simulink model "IonSatSimulationF_UKF"  (R2020b)
settings: Solver=ode3  StartTime=0.0  StopTime=t_sim  FixedStep=TimeStep  MaxStep=30  MinStep=.1  RelTol=1e-3
model workspace (MAT data in the model file):
  repartition_matrix : Simulink.Parameter (value not decoded)
  wheel_number : Simulink.Parameter (value not decoded)
values from neighbouring files (symbols this model uses):
  controller = 1    [Scenario1_Monte_Carlo.m]    (also in main_ADCS_v2.m)
  K = [0.00053417  0  0  0.0070506  0  0 ... (first row only)    [Full_model_PID_MEKF_Scenario3_Monte_Carlo.m]    (also in Full_model_PID_UKF_Scenario1_Monte_Carlo.m; Scenario1_Monte_Carlo.m; main_ADCS_v2.m)
  MODE = 4    [Full_model_PID_MEKF_Scenario1_Monte_Carlo.m]    (also in Full_model_PID_MEKF_Scenario3_Monte_Carlo.m = MODE_SEQUENCE(1); Full_model_PID_UKF_Scenario1_Monte_Carlo.m; Full_model_PID_UKF_Scenario2_Monte_Carlo.m = 2; Full_model_PID_UKF_Scenario3_Monte_Carlo.m = MODE_SEQUENCE(1))
  Use_IGRF = 1    [Full_model_PID_MEKF_Scenario1_Monte_Carlo.m]    (also in Full_model_PID_MEKF_Scenario3_Monte_Carlo.m; Full_model_PID_UKF_Scenario1_Monte_Carlo.m; Full_model_PID_UKF_Scenario2_Monte_Carlo.m; Full_model_PID_UKF_Scenario3_Monte_Carlo.m)
  Use_IGRF_KF = 1    [Full_model_PID_MEKF_Scenario1_Monte_Carlo.m]    (also in Full_model_PID_MEKF_Scenario3_Monte_Carlo.m; Full_model_PID_UKF_Scenario1_Monte_Carlo.m; Full_model_PID_UKF_Scenario2_Monte_Carlo.m; Full_model_PID_UKF_Scenario3_Monte_Carlo.m)
undefined symbols (not defined in the file or in its folder): att, date, deg, DiscIntNeverNeededParam, IonSataero, km, m, orbit, rad, s, sat
libraries: aerolibutil x29, vrlib x22, aerolibconvert2 x14, dspmathops x13, sharedtransform x12, simulink x9, DipoleModel x3, aerolibobsolete x3, sharedutil x3, simulink_extras x2, aerolibcelestial x2, dspstat3 x1
(part 4 of 4)

== system IonSatSimulationF_UKF/Attitude Controller/RW power // saturation/RW1 saturation time counter/If Action Subsystem4 ==
  In1 : Inport
  Action Port : ActionPort  ActionPortLabel=else
  Out1 : Outport  VectorParamsAs1DForOutWhenUnconnected=off
  wires:
  In1/1 -> Out1/1

== system IonSatSimulationF_UKF/Attitude Controller/RW power // saturation/RW1 saturation time counter/If Action Subsystem6 ==
  In1 : Inport
  Action Port : ActionPort  ActionPortLabel=elseif(u1 <= -5999)
  Add : Sum
  Unit Delay : UnitDelay  SampleTime=-1  HasFrameUpgradeWarning=on
  Out1 : Outport  VectorParamsAs1DForOutWhenUnconnected=off
  wires:
  Unit Delay/1 -> Add/2
  Add/1 -> Out1/1, Unit Delay/1
  In1/1 -> Add/1

== system IonSatSimulationF_UKF/Attitude Controller/RW power // saturation/RW2 saturation time counter/If Action Subsystem4 ==
  In1 : Inport
  Action Port : ActionPort  ActionPortLabel=else
  Out1 : Outport  VectorParamsAs1DForOutWhenUnconnected=off
  wires:
  In1/1 -> Out1/1

== system IonSatSimulationF_UKF/Attitude Controller/RW power // saturation/RW2 saturation time counter/If Action Subsystem5 ==
  In1 : Inport
  Action Port : ActionPort  ActionPortLabel=if(u1 >= 5999)
  Add : Sum
  Unit Delay : UnitDelay  SampleTime=-1  HasFrameUpgradeWarning=on
  Out1 : Outport  VectorParamsAs1DForOutWhenUnconnected=off
  wires:
  In1/1 -> Add/1
  Add/1 -> Unit Delay/1, Out1/1
  Unit Delay/1 -> Add/2

== system IonSatSimulationF_UKF/Attitude Controller/RW power // saturation/RW2 saturation time counter/If Action Subsystem6 ==
  In1 : Inport
  Action Port : ActionPort  ActionPortLabel=elseif(u1 <= -5999)
  Add : Sum
  Unit Delay : UnitDelay  SampleTime=-1  HasFrameUpgradeWarning=on
  Out1 : Outport  VectorParamsAs1DForOutWhenUnconnected=off
  wires:
  Unit Delay/1 -> Add/2
  Add/1 -> Out1/1, Unit Delay/1
  In1/1 -> Add/1

== system IonSatSimulationF_UKF/Attitude Controller/RW power // saturation/RW3 saturation time counter/If Action Subsystem4 ==
  In1 : Inport
  Action Port : ActionPort  ActionPortLabel=else
  Out1 : Outport  VectorParamsAs1DForOutWhenUnconnected=off
  wires:
  In1/1 -> Out1/1

== system IonSatSimulationF_UKF/Attitude Controller/RW power // saturation/RW3 saturation time counter/If Action Subsystem5 ==
  In1 : Inport
  Action Port : ActionPort  ActionPortLabel=if(u1 >= 5999)
  Add : Sum
  Unit Delay : UnitDelay  SampleTime=-1  HasFrameUpgradeWarning=on
  Out1 : Outport  VectorParamsAs1DForOutWhenUnconnected=off
  wires:
  In1/1 -> Add/1
  Add/1 -> Unit Delay/1, Out1/1
  Unit Delay/1 -> Add/2

== system IonSatSimulationF_UKF/Attitude Controller/RW power // saturation/RW3 saturation time counter/If Action Subsystem6 ==
  In1 : Inport
  Action Port : ActionPort  ActionPortLabel=elseif(u1 <= -5999)
  Add : Sum
  Unit Delay : UnitDelay  SampleTime=-1  HasFrameUpgradeWarning=on
  Out1 : Outport  VectorParamsAs1DForOutWhenUnconnected=off
  wires:
  Unit Delay/1 -> Add/2
  Add/1 -> Out1/1, Unit Delay/1
  In1/1 -> Add/1

== system IonSatSimulationF_UKF/Attitude Controller/RW power // saturation/RW4 saturation time counter/If Action Subsystem4 ==
  In1 : Inport
  Action Port : ActionPort  ActionPortLabel=else
  Out1 : Outport  VectorParamsAs1DForOutWhenUnconnected=off
  wires:
  In1/1 -> Out1/1

== system IonSatSimulationF_UKF/Attitude Controller/RW power // saturation/RW4 saturation time counter/If Action Subsystem5 ==
  In1 : Inport
  Action Port : ActionPort  ActionPortLabel=if(u1 >= 5999)
  Add : Sum
  Unit Delay : UnitDelay  SampleTime=-1  HasFrameUpgradeWarning=on
  Out1 : Outport  VectorParamsAs1DForOutWhenUnconnected=off
  wires:
  In1/1 -> Add/1
  Add/1 -> Unit Delay/1, Out1/1
  Unit Delay/1 -> Add/2

== system IonSatSimulationF_UKF/Attitude Controller/RW power // saturation/RW4 saturation time counter/If Action Subsystem6 ==
  In1 : Inport
  Action Port : ActionPort  ActionPortLabel=elseif(u1 <= -5999)
  Add : Sum
  Unit Delay : UnitDelay  SampleTime=-1  HasFrameUpgradeWarning=on
  Out1 : Outport  VectorParamsAs1DForOutWhenUnconnected=off
  wires:
  Unit Delay/1 -> Add/2
  Add/1 -> Out1/1, Unit Delay/1
  In1/1 -> Add/1

== system IonSatSimulationF_UKF/Uncented Kalman Filter/IGRF Computation block orig/Obtain B_ECI/Dipole Subsystem ==
  In1 : Inport
  Action Port : ActionPort
  Bus Selector1 : BusSelector  OutputSignals=h,lat,long,DCM_i2e
  Dipole Model : DipoleModel/Dipole Model  SystemSampleTime=-1  VariantActivationTime=update diagram  Latency=0  AutoFrameSizeCalculation=off
  Out1 : Outport  VectorParamsAs1DForOutWhenUnconnected=off
  wires:
  In1/1 -> Bus Selector1/1
  Bus Selector1/3 -> Dipole Model/3  "<long>"
  Dipole Model/1 -> Out1/1
  Bus Selector1/1 -> Dipole Model/1  "<h>"
  Bus Selector1/2 -> Dipole Model/2  "<lat>"
  Bus Selector1/4 -> Dipole Model/4  "<DCM_i2e>"

== system IonSatSimulationF_UKF/Uncented Kalman Filter/IGRF Computation block orig/Obtain B_ECI/IGRF Subsystem ==
  In1 : Inport
  Action Port : ActionPort
  Bus Selector : BusSelector  OutputSignals=DCM_i2e,h,lat,long,signal4
  International Geomagnetic Reference Field 12 : aerolibobsolete/International Geomagnetic Reference Field 12  units=Metric (MKS)  time_in=on  month=January  day=1  year=2020  action=None  sv_out=on
      settings: SourceProductBaseCode=AE
  T to nT : Gain  Gain=1E-9
  Terminator{1..9} (9 alike) : Terminator
  Out1 : Outport  VectorParamsAs1DForOutWhenUnconnected=off
  wires:
  In1/1 -> Bus Selector/1
  Bus Selector/2 -> International Geomagnetic Reference Field 12/1  "<h>"
  T to nT/1 -> Out1/1
  Bus Selector/5 -> International Geomagnetic Reference Field 12/4  "<signal4>"
  Bus Selector/4 -> International Geomagnetic Reference Field 12/3  "<long>"
  Bus Selector/3 -> International Geomagnetic Reference Field 12/2  "<lat>"
  International Geomagnetic Reference Field 12/2 -> Terminator1/1
  International Geomagnetic Reference Field 12/10 -> Terminator9/1
  International Geomagnetic Reference Field 12/4 -> Terminator3/1
  International Geomagnetic Reference Field 12/5 -> Terminator4/1
  International Geomagnetic Reference Field 12/3 -> Terminator2/1
  International Geomagnetic Reference Field 12/6 -> Terminator5/1
  International Geomagnetic Reference Field 12/8 -> Terminator7/1
  International Geomagnetic Reference Field 12/7 -> Terminator6/1
  International Geomagnetic Reference Field 12/9 -> Terminator8/1
  International Geomagnetic Reference Field 12/1 -> T to nT/1

== system IonSatSimulationF_UKF/Uncented Kalman Filter/IGRF Computation block1/Obtain B_ECI/Dipole Subsystem ==
  In1 : Inport
  Action Port : ActionPort  ActionPortLabel=else
  Bus Selector1 : BusSelector  OutputSignals=h,lat,long,DCM_i2e
  Dipole Model : DipoleModel/Dipole Model  SystemSampleTime=-1  VariantActivationTime=update diagram  Latency=0  AutoFrameSizeCalculation=off
  Out1 : Outport  VectorParamsAs1DForOutWhenUnconnected=off
  wires:
  In1/1 -> Bus Selector1/1
  Bus Selector1/3 -> Dipole Model/3  "<long>"
  Dipole Model/1 -> Out1/1
  Bus Selector1/1 -> Dipole Model/1  "<h>"
  Bus Selector1/2 -> Dipole Model/2  "<lat>"
  Bus Selector1/4 -> Dipole Model/4  "<DCM_i2e>"

== system IonSatSimulationF_UKF/Uncented Kalman Filter/IGRF Computation block1/Obtain B_ECI/IGRF Subsystem ==
  In1 : Inport
  Action Port : ActionPort  ActionPortLabel=if(u1 > 0)
  Bus Selector : BusSelector  OutputSignals=DCM_i2e,h,lat,long,signal4
  International Geomagnetic Reference Field 12 : aerolibobsolete/International Geomagnetic Reference Field 12  units=Metric (MKS)  time_in=on  month=January  day=1  year=2020  action=None  sv_out=on
      settings: SourceProductBaseCode=AE
  Mux : Mux  Inputs=3
  NED to ECEF : MATLABFcn  MATLABFcn=NED2ecef  OutputDimensions=[3;1]  Output1D=off
  Permute Dimensions : PermuteDimensions
  Product : Product  Multiplication=Matrix(*)
  T to nT : Gain  Gain=1E-9
  Terminator{1..9} (9 alike) : Terminator
  Out1 : Outport  VectorParamsAs1DForOutWhenUnconnected=off
  wires:
  In1/1 -> Bus Selector/1
  Bus Selector/2 -> International Geomagnetic Reference Field 12/1  "<h>"
  T to nT/1 -> Out1/1
  Bus Selector/5 -> International Geomagnetic Reference Field 12/4  "<signal4>"
  Bus Selector/4 -> Mux/3, International Geomagnetic Reference Field 12/3  "<long>"
  Bus Selector/3 -> Mux/2, International Geomagnetic Reference Field 12/2  "<lat>"
  International Geomagnetic Reference Field 12/2 -> Terminator1/1
  International Geomagnetic Reference Field 12/10 -> Terminator9/1
  International Geomagnetic Reference Field 12/4 -> Terminator3/1
  International Geomagnetic Reference Field 12/5 -> Terminator4/1
  International Geomagnetic Reference Field 12/3 -> Terminator2/1
  International Geomagnetic Reference Field 12/1 -> Mux/1
  International Geomagnetic Reference Field 12/6 -> Terminator5/1
  International Geomagnetic Reference Field 12/8 -> Terminator7/1
  International Geomagnetic Reference Field 12/7 -> Terminator6/1
  International Geomagnetic Reference Field 12/9 -> Terminator8/1
  Bus Selector/1 -> Permute Dimensions/1  "<DCM_i2e>"
  Permute Dimensions/1 -> Product/1
  Product/1 -> T to nT/1
  Mux/1 -> NED to ECEF/1
  NED to ECEF/1 -> Product/2

== system IonSatSimulationF_UKF/Uncented Kalman Filter/Sat Attitude/6DOF in ECI frame/Compute Q_ECI ==
  note: https://arxiv.org/pdf/0811.2889.pdf
      | $ω = 2q^*\frac{dq}{dt}$ (13)
      |
      | $\frac{dq}{dt} = \frac{1}{2} q * ω$ (14)
  <Q_ECI> : Inport
  Omega_body : Inport  Port=2
  Gain : Gain  Gain=1/2
  Ground : Ground
  Mux : Mux  Inputs=2
  Quaternion Multiplication : aerolibutil/Quaternion Multiplication
  Quaternion Normalize : sharedutil/Quaternion Normalize  aMode=aMode
      settings: SourceProductBaseCode=AE,PW,DR,MT,UV,VE
  Sum : Sum  Inputs=|++
  dt : Gain
  Q_ECI : Outport  VectorParamsAs1DForOutWhenUnconnected=off
  wires:
  Quaternion Multiplication/1 -> Gain/1
  Omega_body/1 -> Mux/2
  Ground/1 -> Mux/1
  Mux/1 -> Quaternion Multiplication/2
  Quaternion Normalize/1 -> Q_ECI/1  "Q_ECI"
  Sum/1 -> Quaternion Normalize/1
  <Q_ECI>/1 -> Quaternion Multiplication/1, Sum/1
  Gain/1 -> dt/1  "dQ"
  dt/1 -> Sum/2

== system IonSatSimulationF_UKF/Uncented Kalman Filter/Sat Attitude/Magnetorquer physics/Magnétocoupleur 1 ==
  note: les grounds représentant les limites en
      |  moment magnétique du magnétocoupleur (lié à l'intensité)
      | A définir
  m_in (scalar) : Inport
  Constant1 : Constant  Value=sat.mag_t.max_mm1
  Constant2 : Constant  Value=- sat.mag_t.max_mm1
  Constant6 : Constant  Value=sat.mag_t.axe1
  Product : Product
  Saturation Dynamic : simulink/Discontinuities/Saturation Dynamic  OutMin=[]  OutMax=[]  OutDataTypeStr=Inherit: Same as second input  OutDataType=fixdt(1, 16)  OutScaling=2^-10  DoSatur=off
  m_out (vect) : Outport  VectorParamsAs1DForOutWhenUnconnected=off
  wires:
  m_in (scalar)/1 -> Saturation Dynamic/2
  Constant2/1 -> Saturation Dynamic/3
  Constant1/1 -> Saturation Dynamic/1
  Saturation Dynamic/1 -> Product/1
  Product/1 -> m_out (vect)/1
  Constant6/1 -> Product/2

== system IonSatSimulationF_UKF/Uncented Kalman Filter/Sat Attitude/Magnetorquer physics/Magnétocoupleur 2 ==
  note: les grounds représentant les limites en
      |  moment magnétique du magnétocoupleur (lié à l'intensité)
      | A définir
  m_in (scalar) : Inport
  Constant : Constant  Value=- sat.mag_t.max_mm2
  Constant1 : Constant  Value=sat.mag_t.max_mm2
  Constant6 : Constant  Value=sat.mag_t.axe2
  Product : Product
  Saturation Dynamic : simulink/Discontinuities/Saturation Dynamic  OutMin=[]  OutMax=[]  OutDataTypeStr=Inherit: Same as second input  OutDataType=fixdt(1, 16)  OutScaling=2^-10  DoSatur=off
  m_out (vect) : Outport  VectorParamsAs1DForOutWhenUnconnected=off
  wires:
  m_in (scalar)/1 -> Saturation Dynamic/2
  Constant/1 -> Saturation Dynamic/3
  Constant1/1 -> Saturation Dynamic/1
  Product/1 -> m_out (vect)/1
  Constant6/1 -> Product/2
  Saturation Dynamic/1 -> Product/1

== system IonSatSimulationF_UKF/Uncented Kalman Filter/Sat Attitude/Magnetorquer physics/Magnétocoupleur 3 ==
  note: les grounds représentant les limites en
      |  moment magnétique du magnétocoupleur (lié à l'intensité)
      | A définir
  m_in (scalar) : Inport
  Constant1 : Constant  Value=sat.mag_t.max_mm3
  Constant2 : Constant  Value=- sat.mag_t.max_mm3
  Constant6 : Constant  Value=sat.mag_t.axe3
  Product : Product
  Saturation Dynamic : simulink/Discontinuities/Saturation Dynamic  OutMin=[]  OutMax=[]  OutDataTypeStr=Inherit: Same as second input  OutDataType=fixdt(1, 16)  OutScaling=2^-10  DoSatur=off
  m_out (vect) : Outport  VectorParamsAs1DForOutWhenUnconnected=off
  wires:
  m_in (scalar)/1 -> Saturation Dynamic/2
  Constant2/1 -> Saturation Dynamic/3
  Constant1/1 -> Saturation Dynamic/1
  Product/1 -> m_out (vect)/1
  Constant6/1 -> Product/2
  Saturation Dynamic/1 -> Product/1

== matlab function IonSatSimulationF_UKF/Disturbance Torques/Aerodynamic Model/Calculate - Az & El Angle/MATLAB Function ==
  data: x input; elevation output; y input; z input
function elevation = fcn(x,y,z)

elevation = z/sqrt(x^2 + y^2 + z^2);

== matlab function IonSatSimulationF_UKF/Reference/q_retrograde/"Avoids" sign change should be improved/MATLAB Function ==
  data: u1 input; y output; u2 input
function y  = fcn(u1, u2)
s=dot(sign(u1),sign(u2));
if sign(s)<0
    y=1;
else
    y=0;
end
end

== matlab function IonSatSimulationF_UKF/Reference/q_retrograde/"Avoids" sign change should be improved/MATLAB Function1 ==
  data: u input; y output
function y = fcn(u)

y = mod(u,2);

== matlab function IonSatSimulationF_UKF/Reference/q_drag/"Avoids" sign change should be improved/MATLAB Function ==
  data: u1 input; y output; u2 input
function y  = fcn(u1, u2)
s=dot(sign(u1),sign(u2));
if sign(s)<0
    y=1;
else
    y=0;
end
end

== matlab function IonSatSimulationF_UKF/Reference/q_drag/"Avoids" sign change should be improved/MATLAB Function1 ==
  data: u input; y output
function y = fcn(u)

y = mod(u,2);

== matlab function IonSatSimulationF_UKF/Reference/q_sun_sun/"Avoids" sign change should be improved/MATLAB Function ==
  data: u1 input; y output; u2 input
function y  = fcn(u1, u2)
s=dot(sign(u1),sign(u2));
if sign(s)<0
    y=1;
else
    y=0;
end
end

== matlab function IonSatSimulationF_UKF/Time propagator/MATLAB Function ==
  data: t input; Y output; DOY output; S output
function [Y, DOY, S] = DOY(t)
Y = 2022 + fix(t/31557600);
DOY = 1+fix((t-floor(t/31557600)*31557600)/86400);
S = t - fix(t/31557600)*31557600 - (DOY-1)*86400;

== matlab function IonSatSimulationF_UKF/Reference/q_sun_sun/"Avoids" sign change should be improved/MATLAB Function1 ==
  data: u input; y output
function y = fcn(u)

y = mod(u,2);

== matlab function IonSatSimulationF_UKF/Reference/q_sun_aero/"Avoids" sign change should be improved/MATLAB Function ==
  data: u1 input; y output; u2 input
function y  = fcn(u1, u2)
s=dot(sign(u1),sign(u2));
if sign(s)<0
    y=1;
else
    y=0;
end
end

== matlab function IonSatSimulationF_UKF/Reference/q_sun_aero/"Avoids" sign change should be improved/MATLAB Function1 ==
  data: u input; y output
function y = fcn(u)

y = mod(u,2);

== matlab function IonSatSimulationF_UKF/Reference/q_sun_drag/"Avoids" sign change should be improved/MATLAB Function ==
  data: u1 input; y output; u2 input
function y  = fcn(u1, u2)
s=dot(sign(u1),sign(u2));
if sign(s)<0
    y=1;
else
    y=0;
end
end

== matlab function IonSatSimulationF_UKF/Reference/q_sun_drag/"Avoids" sign change should be improved/MATLAB Function1 ==
  data: u input; y output
function y = fcn(u)

y = mod(u,2);

== matlab function IonSatSimulationF_UKF/Attitude Controller/RW power // saturation/Steady state Power consumption ==
  data: RW1 input; WP1 output; RW2 input; RW3 input; RW4 input; WP2 output; WP3 output; WP4 output
function [WP1,WP2,WP3,WP4] = fcn(RW1,RW2,RW3,RW4)

WP1 = 0.1414*RW1 - 68.988;
WP2 = 0.1414*RW2 - 68.988;
WP3 = 0.1414*RW3 - 68.988;
WP4 = 0.1414*RW4 - 68.988;

== matlab function IonSatSimulationF_UKF/Uncented Kalman Filter/IGRF Computation block orig/ECI To LLA ==
  data: X_ECEF input; h output; lat output; long output
function [h, lat, long] = fcn(X_ECEF)
    h = 0;
    lat = 0;
    long = 0;
[lat, long, h] = ecef2geod(X_ECEF(1),X_ECEF(2),X_ECEF(3));

== matlab function IonSatSimulationF_UKF/Reference/q_orbital/"Avoids" sign change should be improved/MATLAB Function ==
  data: u1 input; y output; u2 input
function y  = fcn(u1, u2)
s=dot(sign(u1),sign(u2));
if sign(s)<0
    y=1;
else
    y=0;
end
end

== matlab function IonSatSimulationF_UKF/Reference/q_orbital/"Avoids" sign change should be improved/MATLAB Function1 ==
  data: u input; y output
function y = fcn(u)

y = mod(u,2);

== matlab function IonSatSimulationF_UKF/Initialize Function/orb2rv ==
  data: a input; r output; e input; i input; O input; o input; nu input; v output; truLon input; argLat input; lonPer input
%----------------------- Begin Code Sequence -----------------------------%
% Purpose:                                                                %
% Convert a given set of Keplerian Orbital Elements to state vectors in   %
% in the ECI frame of reference                                           %
%                                                                         %
%-------------------------------------------------------------------------%
%                                                                         %
% Inputs:                                                                 %
%-------- 
%a                      [1 x N]                         Semimajor axis
%                                                       (km)
%
%e                      [1 x N]                         Eccentricity Magnitude
%                                                       (unitless)
%
%i                      [1 x N]                         inclination
%                                                       (radians)
%
%O                      [1 x N]                         Right Ascention of
%                                                       the ascending node
%                                                       (radians)
%
%o                      [1 x N]                         Argument of perigee
%                                                       (radians)
%
%nu                     [1 x N]                         True Anomaly
%                                                       (radians)
%
%truLon                 [1 x N]                         True Longitude
%                                                       (radians)
%
%argLat                 [1 x N]                         Argument of Latitude
%                                                       (radians)
%
%lonPer                 [1 x N]                         Longitude of Periapse
%                                                       (radians)
%
%mu                     double                          Gravitational Constant
%                                                       Defaults to Earth if
%                                                       not specified
%
% Outputs:
%---------                                                                %
%r_ECI                  [3 x N]                         Position Vector in
%                                                       ECI coordinate
%                                                       frame of reference
%
%v_ECI                  [3 x N]                         Velocity vector in
%                                                       ECI coordinate
%                                                       frame of reference
%
% References:
%-------------
%Vallado,D. Fundamentals of Astrodynamics and Applications. 2007.
%
% Function Dependencies:
%------------------
%None
%------------------------------------------------------------------       %
% Programed by Darin Koblick  03-04-2012                                  %
%------------------------------------------------------------------       %
function [r,v] = orb2rv(a,e,i,O,o,nu,truLon,argLat,lonPer)
mu = 398600.4418;
%Make all inputs consistent w/ dimensions
a = a(:); e = e(:); i = i(:); O = O(:); o = o(:); nu = nu(:);
if e<1
    p=a*(1-e*e);
else
    p=2*a;
end
ietol = 1e-8;
idx = e < ietol & mod(i,pi) < ietol;
if any(idx); o(idx) = 0; O(idx) = 0; nu(idx) = truLon(idx); end
idx = e < ietol & mod(i,pi) > ietol;
if any(idx); o(idx) = 0; nu(idx) = argLat(idx); end
idx = e > ietol & mod(i,pi) < ietol;
if any(idx); O(idx) = 0; o(idx) = lonPer(idx); end
%Find rPQW and vPQW
rPQW = cat(2,p.*cos(nu)./(1 +e.*cos(nu)),p.*sin(nu)./(1+e.*cos(nu)),zeros(size(nu)));
vPQW = cat(2,-sqrt(mu./p).*sin(nu),sqrt(mu./p).*(e+cos(nu)),zeros(size(nu)));
%Create Transformation Matrix
PQW2IJK = NaN(3,3,size(p,1));
cO = cos(O); sO = sin(O); co = cos(o); so = sin(o); ci = cos(i); si = sin(i);
PQW2IJK(1,1,:) = cO.*co-sO.*so.*ci; PQW2IJK(1,2,:) = -cO.*so-sO.*co.*ci; PQW2IJK(1,3,:) = sO.*si;
PQW2IJK(2,1,:) = sO.*co+cO.*so.*ci; PQW2IJK(2,2,:) = -sO.*so+cO.*co.*ci; PQW2IJK(2,3,:) = -cO.*si;
PQW2IJK(3,1,:) = so.*si;            PQW2IJK(3,2,:) = co.*si;             PQW2IJK(3,3,:) = ci;
%Transform rPQW and vPQW to rECI and vECI
r = multiDimMatrixMultiply(PQW2IJK,rPQW)';  
v = multiDimMatrixMultiply(PQW2IJK,vPQW)';
end
function c = multiDimMatrixMultiply(a,b)
c = NaN(size(b));
c(:,1) = sum(bsxfun(@times,a(1,:,:),permute(b,[3 2 1])),2);
c(:,2) = sum(bsxfun(@times,a(2,:,:),permute(b,[3 2 1])),2);
c(:,3) = sum(bsxfun(@times,a(3,:,:),permute(b,[3 2 1])),2);
end

== matlab function IonSatSimulationF_UKF/Uncented Kalman Filter/IGRF Computation block1/ECI To LLA ==
  data: X_ECEF input; h output; lat output; long output
function [h, lat, long] = fcn(X_ECEF)
    h = 0;
    lat = 0;
    long = 0;
[lat, long, h] = ecef2geod(X_ECEF(1),X_ECEF(2),X_ECEF(3));

== matlab function IonSatSimulationF_UKF/Disturbance Torques/Aerodynamic Model/Get Density/ECI To LLA ==
  data: X_ECEF input; h output; lat output; long output
function [h, lat, long] = fcn(X_ECEF)
    h = 0;
    lat = 0;
    long = 0;
[lat, long, h] = ecef2geod(X_ECEF(1),X_ECEF(2),X_ECEF(3));

== matlab function IonSatSimulationF_UKF/IGRF Computation block/ECI To LLA ==
  data: X_ECEF input; h output; lat output; long output
function [h, lat, long] = fcn(X_ECEF)
    h = 0;
    lat = 0;
    long = 0;
[lat, long, h] = ecef2geod(X_ECEF(1),X_ECEF(2),X_ECEF(3));

== matlab function IonSatSimulationF_UKF/Disturbance Torques/Aerodynamic Model/Get Density/MATLAB Function2 ==
  data: u input; y output
function y = fcn(u)
y = u(6);

== matlab function IonSatSimulationF_UKF/Time propagator/UTC to JD ==
  data: Time_UTC input; JD output
function JD = fcn(Time_UTC)

% JD = juliandate(Time_UTC);
JD = Dt2jD(Time_UTC);

== matlab function IonSatSimulationF_UKF/Time propagator/JD to UTC ==
  data: JD input; Time_UTC output
function Time_UTC = fcn(JD)
    coder.extrinsic('datetime','datevec');
    Time_UTC = [0,0,0,0,0,0];
Time_UTC =  datevec(datetime(JD,'convertfrom','juliandate'));

== matlab function IonSatSimulationF_UKF/Thruster activation/MATLAB Function ==
  data: u input; y output
function y = fcn(u)
% t0 less or equal than waiting time between 2 thrusts
% or 
% sat.thruster.firstimpulse <= sat.thruster.wait

time=u(1);
duration=u(2);
t0=u(3);
wait=u(4);
N=u(5)-1;
boolean=0;
booleant=0;

if (time<t0)
    boolean=0;
end

if (time>=t0)
        m=fix(time/(duration+wait));
        if (m<=N)&&((t0+m*(duration+wait)<time)&&(time<(t0+m*(duration+wait)+duration)))
            boolean=1;
        end
        
end

y = booleant~=boolean;
